simulink model "RC_CircuitSimulation"  (R2022b)
settings: Solver=ode23tb  StartTime=0.0  StopTime=10.0  MaxStep=1e-3  RelTol=1e-3
values from neighbouring files (symbols this model uses):
  C = 1e-4    (= 0.0001)    [RC_CircuitParameters.m]
  R = 1000    [RC_CircuitParameters.m]
libraries: spsRMSLib x1
settings Model: Creator=MOHAMED  LastModifiedBy=MOHAMED

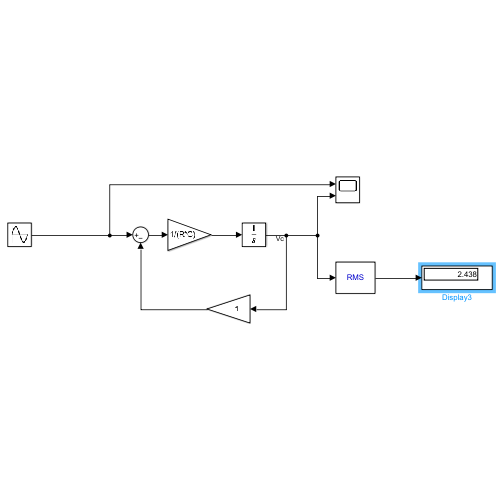
[thumbnail: Simulink's stored preview of the top-level diagram]
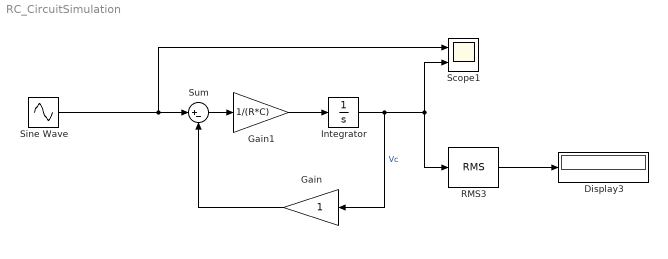
== system RC_CircuitSimulation ==
  Display3 : Display
  Gain : Gain
  Gain1 : Gain  Gain=1/(R*C)
  Integrator : Integrator
  RMS3 : spsRMSLib/RMS  TrueRMS=on  Freq=60  RMSInit=120  Ts=0
  Scope1 : Scope  NumInputPorts=2
  Sine Wave : Sin  Amplitude=5  Frequency=2*pi  SampleTime=0
  Sum : Sum  Inputs=|+-
  wires:
  Sine Wave/1 -> Scope1/1, Sum/1
  Integrator/1 -> Gain/1, RMS3/1, Scope1/2  "Vc"
  Gain1/1 -> Integrator/1
  Sum/1 -> Gain1/1
  Gain/1 -> Sum/2
  RMS3/1 -> Display3/1
